simulink model "completoconesnamblamal"  (R2013a)
settings: Solver=ode45  StartTime=0.0  StopTime=200  RelTol=1e-3
values from neighbouring files (symbols this model uses):
  g = 9.81    [miosinlazoalgebraico.m]    (also in yovalores.m)
  theta1 = (m1*lc1*lc1)+(m2*l1*l1)+I1    (= 0.09775488)    [miosinlazoalgebraico.m]
  theta2 = (m2*lc2*lc2)+I2    (= 0.00775807)    [miosinlazoalgebraico.m]
  theta3 = (m2*l1*l2)    (= 0.0287)    [miosinlazoalgebraico.m]
  theta4 = (m1*lc1)+(m2*l1)    (= 0.495148)    [miosinlazoalgebraico.m]
  theta5 = (m2*lc2)    (= 0.044485)    [miosinlazoalgebraico.m]
undefined symbols (not defined in the file or in its folder): base1, ensamblaje2, Pieza2, Pieza3, RootGround, RootPart
libraries: mblibv1 x14
settings Model: Creator=Daniel  LastModifiedBy=Daniel
settings SimMechanicsCC: VisOnUpdateDiagram=on  VisDuringSimulation=on

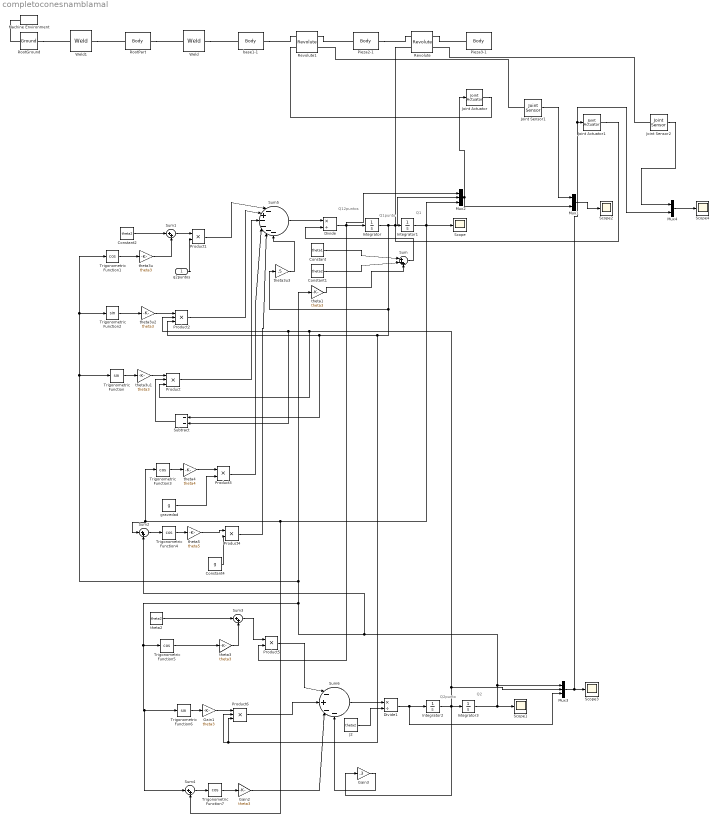
== system completoconesnamblamal ==
  note: Q1
  note: Q1punto
  note: Q12puntos
  note: Q2
  note: Q2punto
  q2puntos : Inport
  Constant : Constant  Value=theta1
  Constant1 : Constant  Value=theta2
  Constant2 : Constant  Value=theta2
  Constant4 : Constant  Value=g
  Divide : Product  Inputs=*/
  Divide1 : Product  Inputs=*/
  Gain1 : Gain  Gain=theta3
  Gain2 : Gain  Gain=theta3
  Gain3 : Gain  Gain=.3
  Integrator : Integrator
  Integrator1 : Integrator  InitialCondition=pi
  Integrator2 : Integrator
  Integrator3 : Integrator  InitialCondition=pi
  J2 : Constant  Value=theta2
  Joint Actuator : mblibv1/Sensors &  Actuators/Joint Actuator  UpdateFromCAD=off  PhysicalDomain=Mechanical  PortType=blob  ActuationStyle=Motion  AngleUnits=deg  ArcVelocityUnits=deg/s  ArcAccelerationUnits=deg/s^2  CoordPositionUnits=m  VelocityUnits=m/s  AccelerationUnits=m/s^2  ForceUnits=N  TorqueUnits=N*m  ActiveIO=on  Width=3  DialogClass=MechanicalActuatorBlock  Primitive=R1  ReferenceFrame=Absolute (World)
  Joint Actuator1 : mblibv1/Sensors &  Actuators/Joint Actuator  UpdateFromCAD=off  PhysicalDomain=Mechanical  PortType=blob  ActuationStyle=Motion  AngleUnits=deg  ArcVelocityUnits=deg/s  ArcAccelerationUnits=deg/s^2  CoordPositionUnits=m  VelocityUnits=m/s  AccelerationUnits=m/s^2  ForceUnits=N  TorqueUnits=N*m  ActiveIO=on  Width=3  DialogClass=MechanicalActuatorBlock  Primitive=R1  ReferenceFrame=Absolute (World)
  Joint Sensor1 : mblibv1/Sensors &  Actuators/Joint Sensor  UpdateFromCAD=off  PhysicalDomain=Mechanical  PortType=blob  Muxed=on  Pose=off  Angle=on  AngleUnits=deg  ArcVelocity=off  ArcVelocityUnits=deg/s  ArcAcceleration=off  ArcAccelerationUnits=deg/s^2  CoordPosition=on  CoordPositionUnits=m  Velocity=off  VelocityUnits=m/s  Acceleration=off  AccelerationUnits=m/s^2  Quaternion=on  QuaternionDT=off  QuaternionDDT=off  QuaternionUnits=off  OutputVector=[1]  ActiveIO=on  Width=1  DialogClass=MechanicalSensorBlock  Primitive=R1  Force=off  ForceUnits=N  Torque=off  TorqueUnits=N*m  ReferenceFrame=Absolute (World)  ReactionSensedSide=Base  ReactionReferenceFrame=Absolute (World)  ReactionForce=off  ReactionForceUnits=N  ReactionMoment=off  ReactionMomentUnits=N*m
  Joint Sensor2 : mblibv1/Sensors &  Actuators/Joint Sensor  UpdateFromCAD=off  PhysicalDomain=Mechanical  PortType=blob  Muxed=on  Pose=off  Angle=on  AngleUnits=deg  ArcVelocity=off  ArcVelocityUnits=deg/s  ArcAcceleration=off  ArcAccelerationUnits=deg/s^2  CoordPosition=on  CoordPositionUnits=m  Velocity=off  VelocityUnits=m/s  Acceleration=off  AccelerationUnits=m/s^2  Quaternion=on  QuaternionDT=off  QuaternionDDT=off  QuaternionUnits=off  OutputVector=[1]  ActiveIO=on  Width=1  DialogClass=MechanicalSensorBlock  Primitive=R1  Force=off  ForceUnits=N  Torque=off  TorqueUnits=N*m  ReferenceFrame=Absolute (World)  ReactionSensedSide=Base  ReactionReferenceFrame=Absolute (World)  ReactionForce=off  ReactionForceUnits=N  ReactionMoment=off  ReactionMomentUnits=N*m
  Machine Environment : mblibv1/Bodies/Machine Environment  PortType=env  PhysicalDomain=Mechanical  DialogTemplateClass=MECH.MachineEnvironment  SyncWhenCopied=off  Gravity=[0 -9.81 0]  GravityUnits=m/s^2  GravityAsSignal=off  Dimensionality=Auto-detect  AnalysisType=Forward dynamics  LinearAssemblyTolerance=1e-3  LinearAssemblyToleranceUnits=m  AngularAssemblyTolerance=1e-3  AngularAssemblyToleranceUnits=rad  ConstraintSolverType=Stabilizing  ConstraintRelTolerance=1e-4  ConstraintAbsTolerance=1e-4  UseRobustSingularityHandling=off  RedundancyAnalysisToleranceType=Automatically select tolerance  RedundancyAnalysisTolerance=1e-14  StatePerturbationType=Fixed  PerturbationSize=1e-5  VisualizeMachine=on  BodyVisualizationType=Use model default body geometries  BodyColorSelMode=Use model default  DefaultBodyColor=[1 0 0]
  Mux1 : Mux  Inputs=2
  Mux2 : Mux  Inputs=3
  Mux3 : Mux  Inputs=3
  Mux4 : Mux  Inputs=2
  Pieza2-1 : mblibv1/Bodies/Body  LConnTagsString=CS3  RConnTagsString=CS2  UpdateFromCAD=on  PMImportedID=Pieza2-1  DialogClass=MechanicalBodyBlock  Mass=0.734204  MassUnits=kg  InertiaUnits=kg*m^2  Inertia=[0.000264247,2.83059e-10,-6.28102e-08;2.83059e-10,0.0127231,5.8833e-11;-6.28102e-08,5.8833e-11,0.0126365]  Shape=Cylinder  ShapeDims=[1 1]  ShapeUnits=m  ShapeUse=false  Density=1  DensityUnits=kg/m^3  DensityUse=false  GraphicsMode=GFXFILE  GraphicsFileName=ensamblaje2 - Pieza2-1.STL  BodyColorSelMode=COLORPALETTE  BodyColor=[0.79216 0.81961 0.93333]  AttachedToCS=CS1  CG=Right$CG$[0.243387 0.00384817 0.55245]$WORLD$WORLD$m$[1 0 0;0 0 -1;0 1 0]$3x3 Transform$rad$WORLD$false$Pieza2-1::CG(AUTOGEN)  WorkingFrames=Right$CS1$[0.0868146 -0.0215 0.5334]$WORLD$WORLD$m$[1 0 0;0 0 -1;0 1 0]$3x3 Transform$rad$WORLD$false$Pieza2-1::CS1(AUTOGEN)#Right$CS2$[0.454137 0.00380573 0.5334]$WORLD$WORLD$m$[1 0 0;0 1 0;0 0 1]$3x3 Transform$rad$WORLD$true$Pieza2-1:-:Pieza3-1::Pieza2-1(AUTOGEN)#Left$CS3$[0.0235964 0.00386825 0.5715]$WORLD$WORLD$m$[1 0 0;0 1 0;0 0 1]$3x3 Transform$rad$WORLD$true$Pieza2-1:-:base1-1::Pieza2-1(AUTOGEN)  CGPos=[0.243387 0.00384817 0.55245]  CGRot=[1 0 0;0 0 -1;0 1 0]  CS0Pos=[]  CS0Rot=[]  CS1Pos=[0.0868146 -0.0215 0.5334]  CS1Rot=[1 0 0;0 0 -1;0 1 0]  CS2Pos=[0.454137 0.00380573 0.5334]  CS2Rot=[1 0 0;0 1 0;0 0 1]  CS3Pos=[0.0235964 0.00386825 0.5715]  CS3Rot=[1 0 0;0 1 0;0 0 1]  CS4Pos=[]  CS4Rot=[]  CS5Pos=[]  CS5Rot=[]  CS6Pos=[]  CS6Rot=[]  CS7Pos=[]  CS7Rot=[]  CS8Pos=[]  CS8Rot=[]  CS9Pos=[]  CS9Rot=[]  CS10Pos=[]  CS10Rot=[]  CS11Pos=[]  CS11Rot=[]  CS12Pos=[]  CS12Rot=[]  CS13Pos=[]  CS13Rot=[]  CS14Pos=[]  CS14Rot=[]  CS15Pos=[]  CS15Rot=[]  CS16Pos=[]  CS16Rot=[]  CS17Pos=[]  CS17Rot=[]  CS18Pos=[]  CS18Rot=[]  CS19Pos=[]  CS19Rot=[]  CS20Pos=[]  CS20Rot=[]
  Pieza3-1 : mblibv1/Bodies/Body  LConnTagsString=CS2  UpdateFromCAD=on  PMImportedID=Pieza3-1  DialogClass=MechanicalBodyBlock  Mass=0.784305  MassUnits=kg  InertiaUnits=kg*m^2  Inertia=[0.000374519,0.000457935,-7.77784e-07;0.000457935,0.0141418,4.97542e-08;-7.77784e-07,4.97542e-08,0.0141799]  Shape=Cylinder  ShapeDims=[1 1]  ShapeUnits=m  ShapeUse=false  Density=1  DensityUnits=kg/m^3  DensityUse=false  GraphicsMode=GFXFILE  GraphicsFileName=ensamblaje2 - Pieza3-1.STL  BodyColorSelMode=COLORPALETTE  BodyColor=[0.792157;0.819608;0.933333]  AttachedToCS=CS1  CG=Right$CG$[0.632017 0.00378637 0.517632]$WORLD$WORLD$m$[1 0 0;0 0 -1;0 1 0]$3x3 Transform$rad$WORLD$false$Pieza3-1::CG(AUTOGEN)  WorkingFrames=Right$CS1$[0.517355 -0.0215625 0.4953]$WORLD$WORLD$m$[1 0 0;0 0 -1;0 1 0]$3x3 Transform$rad$WORLD$false$Pieza3-1::CS1(AUTOGEN)#Left$CS2$[0.454137 0.00380573 0.5334]$WORLD$WORLD$m$[1 0 0;0 1 0;0 0 1]$3x3 Transform$rad$WORLD$true$Pieza2-1:-:Pieza3-1::Pieza3-1(AUTOGEN)  CGPos=[0.632017 0.00378637 0.517632]  CGRot=[1 0 0;0 0 -1;0 1 0]  CS0Pos=[]  CS0Rot=[]  CS1Pos=[0.517355 -0.0215625 0.4953]  CS1Rot=[1 0 0;0 0 -1;0 1 0]  CS2Pos=[0.454137 0.00380573 0.5334]  CS2Rot=[1 0 0;0 1 0;0 0 1]  CS3Pos=[]  CS3Rot=[]  CS4Pos=[]  CS4Rot=[]  CS5Pos=[]  CS5Rot=[]  CS6Pos=[]  CS6Rot=[]  CS7Pos=[]  CS7Rot=[]  CS8Pos=[]  CS8Rot=[]  CS9Pos=[]  CS9Rot=[]  CS10Pos=[]  CS10Rot=[]  CS11Pos=[]  CS11Rot=[]  CS12Pos=[]  CS12Rot=[]  CS13Pos=[]  CS13Rot=[]  CS14Pos=[]  CS14Rot=[]  CS15Pos=[]  CS15Rot=[]  CS16Pos=[]  CS16Rot=[]  CS17Pos=[]  CS17Rot=[]  CS18Pos=[]  CS18Rot=[]  CS19Pos=[]  CS19Rot=[]  CS20Pos=[]  CS20Rot=[]
  Product : Product  Inputs=3
  Product{1,3..5} (4 alike) : Product
  Product2 : Product  Inputs=3
  Product6 : Product  Inputs=3
  Revolute : mblibv1/Joints/Revolute  LConnTagsString=__newl0|SA1  RConnTagsString=__newr0|SA1  UpdateFromCAD=on  PMImportedID=Pieza2-1:-:Pieza3-1  NumSAPorts=2  CutJoint=off  MarkAsCut=off  Primitives=prismatic  PrimitiveProps=R1$World$[0,0,-1]$revolute  DialogClass=JointBlock  R1Axis=[0,0,-1]
  Revolute1 : mblibv1/Joints/Revolute  LConnTagsString=__newl0|SA1  RConnTagsString=__newr0|SA1  UpdateFromCAD=on  PMImportedID=Pieza2-1:-:base1-1  NumSAPorts=2  CutJoint=off  MarkAsCut=off  Primitives=prismatic  PrimitiveProps=R1$World$[0,0,1]$revolute  DialogClass=JointBlock  R1Axis=[0,0,1]
  RootGround : mblibv1/Bodies/Ground  UpdateFromCAD=on  PMImportedID=RootGround  LeftPortType=env  RightPortType=workingframe  PhysicalDomain=Mechanical  DialogClass=GroundBlock  CoordPosition=[0.189096,0.000658845,0.410054]  CoordPositionUnits=m  StateVectorMgrId=1  MachineId=[2 0]  ShowEnvPort=on
  RootPart : mblibv1/Bodies/Body  LConnTagsString=CS3  RConnTagsString=CS2  UpdateFromCAD=on  PMImportedID=ensamblaje2/RootPart  DialogClass=MechanicalBodyBlock  Mass=0  MassUnits=kg  InertiaUnits=kg*m^2  Inertia=[0,0,0;0,0,0;0,0,0]  Shape=Cylinder  ShapeDims=[1 1]  ShapeUnits=m  ShapeUse=false  Density=1  DensityUnits=kg/m^3  DensityUse=false  GraphicsMode=MACHINE_DEFAULT  BodyColorSelMode=MACHINE_DEFAULT  BodyColor=[1;0;0]  AttachedToCS=CS1  CG=Right$CG$[0.189096 0.000658845 0.410054]$WORLD$WORLD$m$[1 0 0;0 1 0;0 0 1]$3x3 Transform$rad$WORLD$false$ensamblaje2/RootPart::CG(AUTOGEN)  WorkingFrames=Right$CS1$[0 0 0]$WORLD$WORLD$m$[1 0 0;0 1 0;0 0 1]$3x3 Transform$rad$WORLD$false$ensamblaje2/RootPart::CS1(AUTOGEN)#Right$CS2$[0.0235964 -0.00139024 0.329313]$WORLD$WORLD$m$[1 0 0;0 1 0;0 0 1]$3x3 Transform$rad$WORLD$true$base1-1:-:ensamblaje2/RootPart::ensamblaje2/RootPart(AUTOGEN)#Left$CS3$[0.189096 0.000658845 0.410054]$WORLD$WORLD$m$[1 0 0;0 1 0;0 0 1]$3x3 Transform$rad$WORLD$true$RootGround:-:ensamblaje2/RootPart::ensamblaje2/RootPart(AUTOGEN)  CGPos=[0.189096 0.000658845 0.410054]  CGRot=[1 0 0;0 1 0;0 0 1]  CS0Pos=[]  CS0Rot=[]  CS1Pos=[0 0 0]  CS1Rot=[1 0 0;0 1 0;0 0 1]  CS2Pos=[0.0235964 -0.00139024 0.329313]  CS2Rot=[1 0 0;0 1 0;0 0 1]  CS3Pos=[0.189096 0.000658845 0.410054]  CS3Rot=[1 0 0;0 1 0;0 0 1]  CS4Pos=[]  CS4Rot=[]  CS5Pos=[]  CS5Rot=[]  CS6Pos=[]  CS6Rot=[]  CS7Pos=[]  CS7Rot=[]  CS8Pos=[]  CS8Rot=[]  CS9Pos=[]  CS9Rot=[]  CS10Pos=[]  CS10Rot=[]  CS11Pos=[]  CS11Rot=[]  CS12Pos=[]  CS12Rot=[]  CS13Pos=[]  CS13Rot=[]  CS14Pos=[]  CS14Rot=[]  CS15Pos=[]  CS15Rot=[]  CS16Pos=[]  CS16Rot=[]  CS17Pos=[]  CS17Rot=[]  CS18Pos=[]  CS18Rot=[]  CS19Pos=[]  CS19Rot=[]  CS20Pos=[]  CS20Rot=[]
  Scope{,1..4} (5 alike) : Scope
      Scope settings: YMin=4.6966  YMax=4.6981
      Scope1 settings: YMin=2.73642  YMax=2.7365
      Scope2 settings: YMin=4.6966  YMax=4.6981  SaveName=ScopeData2
      Scope3 settings: YMin=2.73642  YMax=2.7365  SaveName=ScopeData3
      Scope4 settings: YMin=4.6966  YMax=4.6981  SaveName=ScopeData4
  Subtract : Sum  Inputs=--
  Sum : Sum  Inputs=|+++
  Sum{1..4} (4 alike) : Sum  Inputs=|++
  Sum5 : Sum  Inputs=|-+----
  Sum6 : Sum  Inputs=|-+--
  Trigonometric Function : Trigonometry
  Trigonometric Function{1,3..5,7} (5 alike) : Trigonometry  Operator=cos
  Trigonometric Function2 : Trigonometry
  Trigonometric Function6 : Trigonometry
  Weld : mblibv1/Joints/Weld  LConnTagsString=__newl0  RConnTagsString=__newr0  UpdateFromCAD=on  PMImportedID=base1-1:-:ensamblaje2/RootPart  NumSAPorts=0  CutJoint=off  MarkAsCut=off  Primitives=weld  PrimitiveProps=W$WORLD$[0.57735,0.57735,0.57735]$weld  DialogClass=JointBlock  WAxis=[0.57735,0.57735,0.57735]
  Weld1 : mblibv1/Joints/Weld  LConnTagsString=__newl0  RConnTagsString=__newr0  UpdateFromCAD=on  PMImportedID=RootGround:-:ensamblaje2/RootPart  NumSAPorts=0  CutJoint=off  MarkAsCut=off  Primitives=weld  PrimitiveProps=W$WORLD$[0.57735,0.57735,0.57735]$weld  DialogClass=JointBlock  WAxis=[0.57735,0.57735,0.57735]
  base1-1 : mblibv1/Bodies/Body  LConnTagsString=CS2  RConnTagsString=CS3  UpdateFromCAD=on  PMImportedID=base1-1  DialogClass=MechanicalBodyBlock  Mass=2.33985  MassUnits=kg  InertiaUnits=kg*m^2  Inertia=[0.0177947,0,0;0,0.0199651,-0.000145344;0,-0.000145344,0.00389253]  Shape=Cylinder  ShapeDims=[1 1]  ShapeUnits=m  ShapeUse=false  Density=1  DensityUnits=kg/m^3  DensityUse=false  GraphicsMode=GFXFILE  GraphicsFileName=ensamblaje2 - base1-1.STL  BodyColorSelMode=COLORPALETTE  BodyColor=[0.792157;0.819608;0.933333]  AttachedToCS=CS1  CG=Right$CG$[0.0235964 -0.00139024 0.329313]$WORLD$WORLD$m$[1 0 0;0 1 0;0 0 1]$3x3 Transform$rad$WORLD$false$base1-1::CG(AUTOGEN)  WorkingFrames=Right$CS1$[0.0235964 -0.0332157 0.1905]$WORLD$WORLD$m$[1 0 0;0 1 0;0 0 1]$3x3 Transform$rad$WORLD$false$base1-1::CS1(AUTOGEN)#Left$CS2$[0.0235964 -0.00139024 0.329313]$WORLD$WORLD$m$[1 0 0;0 1 0;0 0 1]$3x3 Transform$rad$WORLD$true$base1-1:-:ensamblaje2/RootPart::base1-1(AUTOGEN)#Right$CS3$[0.0235964 0.00386825 0.5715]$WORLD$WORLD$m$[1 0 0;0 1 0;0 0 1]$3x3 Transform$rad$WORLD$true$Pieza2-1:-:base1-1::base1-1(AUTOGEN)  CGPos=[0.0235964 -0.00139024 0.329313]  CGRot=[1 0 0;0 1 0;0 0 1]  CS0Pos=[]  CS0Rot=[]  CS1Pos=[0.0235964 -0.0332157 0.1905]  CS1Rot=[1 0 0;0 1 0;0 0 1]  CS2Pos=[0.0235964 -0.00139024 0.329313]  CS2Rot=[1 0 0;0 1 0;0 0 1]  CS3Pos=[0.0235964 0.00386825 0.5715]  CS3Rot=[1 0 0;0 1 0;0 0 1]  CS4Pos=[]  CS4Rot=[]  CS5Pos=[]  CS5Rot=[]  CS6Pos=[]  CS6Rot=[]  CS7Pos=[]  CS7Rot=[]  CS8Pos=[]  CS8Rot=[]  CS9Pos=[]  CS9Rot=[]  CS10Pos=[]  CS10Rot=[]  CS11Pos=[]  CS11Rot=[]  CS12Pos=[]  CS12Rot=[]  CS13Pos=[]  CS13Rot=[]  CS14Pos=[]  CS14Rot=[]  CS15Pos=[]  CS15Rot=[]  CS16Pos=[]  CS16Rot=[]  CS17Pos=[]  CS17Rot=[]  CS18Pos=[]  CS18Rot=[]  CS19Pos=[]  CS19Rot=[]  CS20Pos=[]  CS20Rot=[]
  gravedad : Constant  Value=g
  theta1 : Gain  Gain=theta3
  theta2 : Constant  Value=theta2
  theta3 : Gain  Gain=theta3
  theta3u : Gain  Gain=theta3
  theta3u1 : Gain  Gain=theta3
  theta3u2 : Gain  Gain=theta3
  theta3u3 : Gain  Gain=.5
  theta4 : Gain  Gain=theta4
  theta5 : Gain  Gain=theta5
  wires:
  Constant2/1 -> Sum1/1
  theta3u/1 -> Sum1/2
  Trigonometric Function1/1 -> theta3u/1
  Sum1/1 -> Product1/1
  q2puntos/1 -> Product1/2
  Product1/1 -> Sum5/1
  Trigonometric Function2/1 -> theta3u2/1
  theta3u2/1 -> Product2/1
  Product2/1 -> Sum5/2
  Product/1 -> Sum5/3
  Trigonometric Function/1 -> theta3u1/1
  theta3u1/1 -> Product/1
  Product3/1 -> Sum5/4
  Trigonometric Function3/1 -> theta4/1
  theta4/1 -> Product3/1
  gravedad/1 -> Product3/2
  Product4/1 -> Sum5/5
  Trigonometric Function4/1 -> theta5/1
  Sum2/1 -> Trigonometric Function4/1
  theta5/1 -> Product4/1
  Constant4/1 -> Product4/2
  Trigonometric Function5/1 -> theta3/1
  theta2/1 -> Sum3/1
  theta3/1 -> Sum3/2
  Sum3/1 -> Product5/1
  Divide/1 -> Mux2/1, Product5/2, Integrator/1
  Product5/1 -> Sum6/1
  Trigonometric Function6/1 -> Gain1/1
  Product6/1 -> Sum6/2
  Integrator/1 -> Mux2/2, Integrator1/1, theta3u3/1, Product6/3, Product6/2, Subtract/1, Product2/3
  Gain1/1 -> Product6/1
  Gain2/1 -> Sum6/3
  Integrator3/1 -> Mux3/1, Sum2/2, theta1/1, Trigonometric Function/1, Trigonometric Function2/1, Trigonometric Function1/1, Sum4/1, Trigonometric Function6/1, Trigonometric Function5/1, Scope1/1
  Trigonometric Function7/1 -> Gain2/1
  Sum4/1 -> Trigonometric Function7/1
  Integrator1/1 -> Mux2/3, Sum4/2, Trigonometric Function3/1, Sum2/1, Scope/1
  Constant/1 -> Sum/1
  Constant1/1 -> Sum/2
  theta1/1 -> Sum/3
  Sum/1 -> Divide/2
  Sum5/1 -> Divide/1
  Sum6/1 -> Divide1/1
  Divide1/1 -> Mux3/3, Integrator2/1
  J2/1 -> Divide1/2
  Subtract/1 -> Product/2
  theta3u3/1 -> Sum5/6
  Gain3/1 -> Sum6/4
  Mux2/1 -> Joint Actuator/1, Mux1/2
  Joint Sensor1/1 -> Mux1/1
  Mux1/1 -> Scope2/1
  Integrator2/1 -> Gain3/1, Mux3/2, Product/3, Subtract/2, Product2/2, Integrator3/1
  Joint Sensor2/1 -> Mux4/1
  Mux3/1 -> Mux4/2, Joint Actuator1/1, Scope3/1
  Mux4/1 -> Scope4/1
  connections:
  RootPart/RConn1 -- Weld/LConn1
  Weld/RConn1 -- base1-1/LConn1
  Pieza2-1/RConn1 -- Revolute/LConn1
  Revolute/RConn1 -- Pieza3-1/LConn1
  base1-1/RConn1 -- Revolute1/LConn1
  Revolute1/RConn1 -- Pieza2-1/LConn1
  RootGround/RConn1 -- Weld1/LConn1
  Weld1/RConn1 -- RootPart/LConn1
  RootGround/LConn1 -- Machine Environment/RConn1
  Joint Actuator/RConn1 -- Revolute1/LConn2
  Joint Sensor1/LConn1 -- Revolute1/RConn2
  Joint Actuator1/RConn1 -- Revolute/LConn2
  Joint Sensor2/LConn1 -- Revolute/RConn2
